simulink model "dinamici"  (R2026a)
settings: Solver=VariableStepAuto
undefined symbols (not defined in the file or in its folder): init
settings Model: Creator=atreyu  LastModifiedBy=atreyu
settings DebuggingCC: UnderSpecifiedDimensionMsg=warning

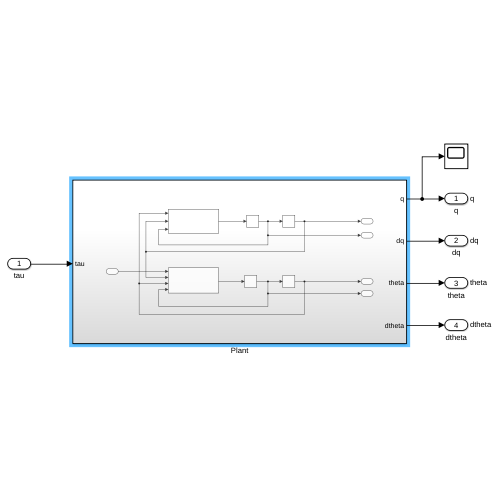
[thumbnail: Simulink's stored preview of the top-level diagram]
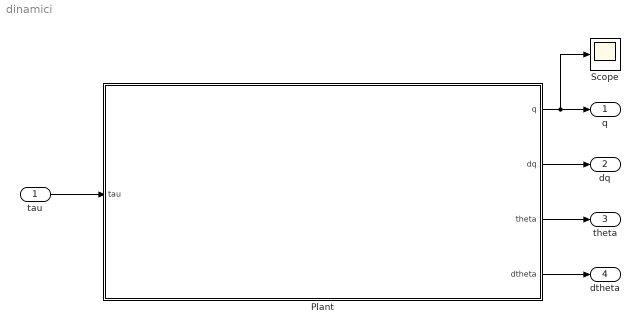
== system dinamici ==
  tau : Inport
  Plant : Subsystem
  Scope : Scope
      settings: ActiveDisplayYMinimum=-10.051020408163266  ActiveDisplayYMaximum=9.94897959183673
  q : Outport  SignalName=q
  dq : Outport  Port=2  SignalName=dq
  theta : Outport  Port=3  SignalName=theta
  dtheta : Outport  Port=4  SignalName=dtheta
  wires:
  Plant/1(q) -> Scope/1, q/1
  Plant/2(dq) -> dq/1
  Plant/3(theta) -> theta/1
  Plant/4(dtheta) -> dtheta/1
  tau/1 -> Plant/1(tau)

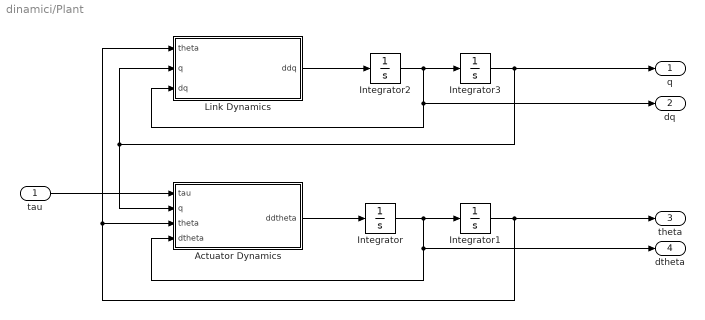
== system dinamici/Plant ==
  tau : Inport
  Actuator Dynamics : MATLAB Function  TreatAsAtomicUnit=on
  Integrator : Integrator  InitialCondition=init.dtheta
  Integrator1 : Integrator  InitialCondition=init.theta
  Integrator2 : Integrator  InitialCondition=init.dq
  Integrator3 : Integrator  InitialCondition=init.q
  Link Dynamics : MATLAB Function  TreatAsAtomicUnit=on
  q : Outport
  dq : Outport  Port=2
  theta : Outport  Port=3
  dtheta : Outport  Port=4
  wires:
  Actuator Dynamics/1(ddtheta) -> Integrator/1
  Integrator3/1 -> q/1, Actuator Dynamics/2(q), Link Dynamics/2(q)
  Integrator/1 -> dtheta/1, Actuator Dynamics/4(dtheta), Integrator1/1
  tau/1 -> Actuator Dynamics/1(tau)
  Link Dynamics/1(ddq) -> Integrator2/1
  Integrator1/1 -> theta/1, Link Dynamics/1(theta), Actuator Dynamics/3(theta)
  Integrator2/1 -> dq/1, Link Dynamics/3(dq), Integrator3/1

== matlab function dinamici/Plant/Actuator Dynamics ==
  data: tau input size=[2 1]; q input size=[2 1]; ddtheta output size=[2 1]; theta input size=[2 1]; dtheta input size=[2 1]; params parameter
function ddtheta = fcn(tau, q, theta, dtheta, params)

ddtheta = tau;
ddtheta = ddtheta - params.K_s*(theta - q);
ddtheta = ddtheta - params.B_m*dtheta;
ddtheta = inv(params.J_m)*ddtheta;
% ddtheta = (tau - params.K_s*(theta - q) - params.B_m*dtheta)/params.J_m;

end

== matlab function dinamici/Plant/Link Dynamics ==
  data: theta input size=[2 1]; q input size=[2 1]; dq input size=[2 1]; ddq output size=[2 1]; params parameter
function ddq = fcn(theta, q, dq, params)

ddq = inv(mass_dynamics(q,params))* ...
        (params.K_s*(theta - q) - ...
        coriolis_dynamics(q,dq,params)*dq - ...
        gravity_dynamics(q,params));

end
